simulink model "cessna_practicemodel"  (R2022a)
settings: Solver=VariableStepAuto  StartTime=0.0  StopTime=10  RelTol=1e-3
undefined symbols (not defined in the file or in its folder): Clat, Clong, DiscIntNeverNeededParam, Kr, Kr_lat, krlat, krlong, Kw, Kw_lat, Kx, Kx_lat, kxlat, kxlong
libraries: airlib x1
settings Model: Creator=steph  LastModifiedBy=steph

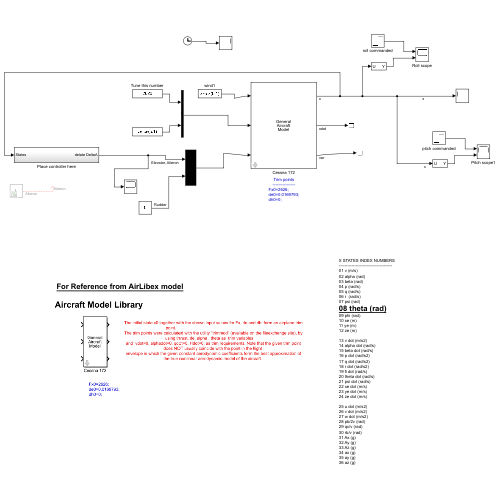
[thumbnail: Simulink's stored preview of the top-level diagram]
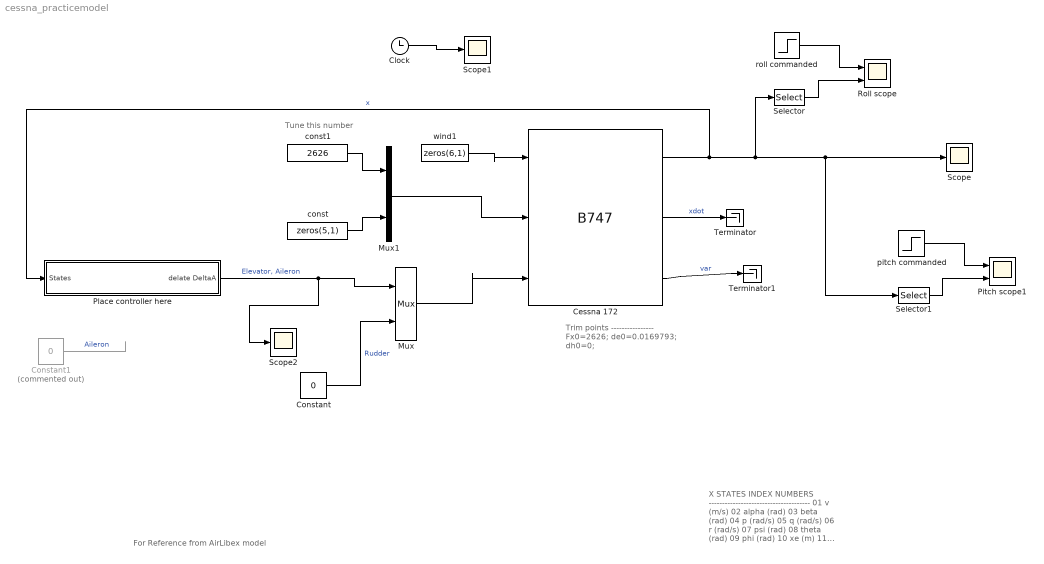
== system cessna_practicemodel ==
  note: For Reference from AirLibex model
  note: X STATES INDEX NUMBERS
      | --------------------------------------
      | 01 v (m/s)
      | 02 alpha (rad)
      | 03 beta (rad)
      | 04 p (rad/s)
      | 05 q (rad/s)
      | 06 r (rad/s)
      | 07 psi (rad)
      | 08 theta (rad)
      | 09 phi (rad)
      | 10 xe (m)
      | 11 ye (m)
      | 12 ze (m)
      |
      | 13 v dot (m/s2)
      | 14 alpha dot (rad/s)
      | 15 beta dot (rad/s)
      | 16 p dot (rad/s2)
      | 17 q dot (rad/s2)
      | 18 r dot (rad/s2)
      | 19 fi dot (rad/s)
      | 20 theta dot (rad/s)
      | 21 psi dot (rad/s)
      | 22 xe dot (m/s)
      | 23 ye dot (m/s)
      | 24 ze dot (m/s)
      |
      | 25 u dot (m/s2)
      | 26 v dot (m/s2)
      | 27 w dot (m/s2)
      | 28 pb/2v (rad)
      | 29 qc/v (rad)
      | 30 rb/v (rad)
      | 31 Ax (g)
      | 32 Ay (g)
      | 33 Az (g)
      | 34 ax (g)
      | 35 ay (g)
      | 36 az (g)
  note: Trim points
      | ----------------
      | Fx0=2626;
      | de0=0.0169793;
      | dh0=0;
  note: Tune this number
  " Cessna 172 " : airlib/B747  GM1="[1.4935  10.9118  16.1651  1285.3  1824.9  2666.9  0 0 0   1043.3]"  CD_wind="[0.031   0.13  0  0.06  0]"  CL_wind="[0.31   5.143    3.9   0.43   0]"  Cm_body="[-0.015  -0.89  -12.4   -1.28   0]"  CY_body="[0  -0.31 -0.037  0.21  0.0  0.187]"  Cl_body="[0    -0.089  -0.47  0.096  -0.178  0.0147]"  Cn_body="[0    0.065    -0.03  -0.099  -0.053  -0.0657]"  x0="[100  -0.0412737 0   0 0 0   0 -0.0412737 0   0 0 60]"
  Clock : Clock
  Constant : Constant  Value=0
  Constant1 : Constant  Commented=on  Value=0
  Mux : Mux  Inputs=2
  Mux1 : Mux  Inputs=[1 5]
  Pitch scope1 : Scope  NumInputPorts=2
  Place controller here : Subsystem
  Roll scope : Scope  NumInputPorts=2
  Scope : Scope
  Scope1 : Scope
  Scope2 : Scope
  Selector : Selector  InputPortWidth=12  IndexOptions=Index vector (dialog)  Indices=[9]  OutputSizes=1
  Selector1 : Selector  InputPortWidth=12  IndexOptions=Index vector (dialog)  Indices=[8]  OutputSizes=1
  Terminator : Terminator
  Terminator1 : Terminator
  const : Constant  Value=zeros(5,1)
  const1 : Constant  Value=2626
  pitch commanded : Step  Time=70  After=15*pi/180  SampleTime=0
  roll commanded : Step  Time=10  After=15*pi/180  SampleTime=0
  wind1 : Constant  Value=zeros(6,1)
  wires:
  " Cessna 172 "/2 -> Terminator/1  "xdot"
  " Cessna 172 "/3 -> Terminator1/1  "var"
  wind1/1 -> " Cessna 172 "/1
  Mux1/1 -> " Cessna 172 "/2
  Mux/1 -> " Cessna 172 "/3
  Place controller here/1(delate DeltaA) -> Scope2/1, Mux/1  "Elevator, Aileron"
  Constant/1 -> Mux/2  "Rudder"
  Constant1/1 -> ?  "Aileron"
  const/1 -> Mux1/2
  const1/1 -> Mux1/1
  Selector/1 -> Roll scope/2
  roll commanded/1 -> Roll scope/1
  " Cessna 172 "/1 -> Place controller here/1(States), Selector/1, Selector1/1, Scope/1  "x"
  Selector1/1 -> Pitch scope1/2
  pitch commanded/1 -> Pitch scope1/1
  Clock/1 -> Scope1/1

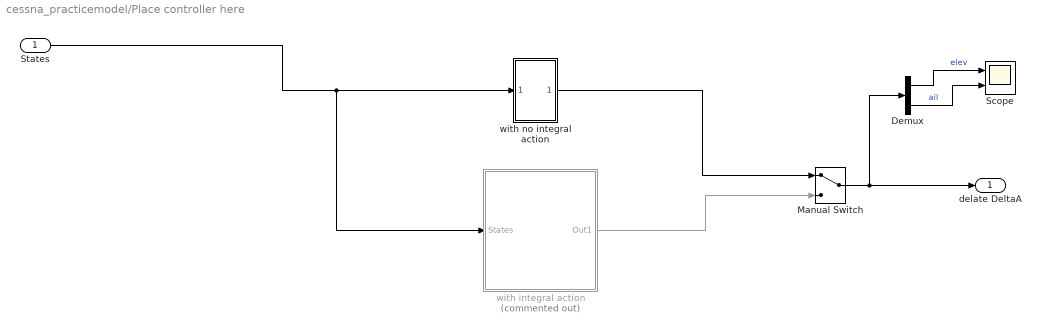
== system cessna_practicemodel/Place controller here ==
  States : Inport
  Demux : Demux  Outputs=2
  Manual Switch : ManualSwitch
  Scope : Scope  NumInputPorts=2
  with integral action : Subsystem  Commented=on
  with no integral action : Subsystem
  delate DeltaA : Outport
  wires:
  States/1 -> with integral action/1(States), with no integral action/1(In1)
  Manual Switch/1 -> Demux/1, delate DeltaA/1
  with no integral action/1(Out1) -> Manual Switch/1
  with integral action/1(Out1) -> Manual Switch/2
  Demux/1 -> Scope/1  "elev"
  Demux/2 -> Scope/2  "ail"

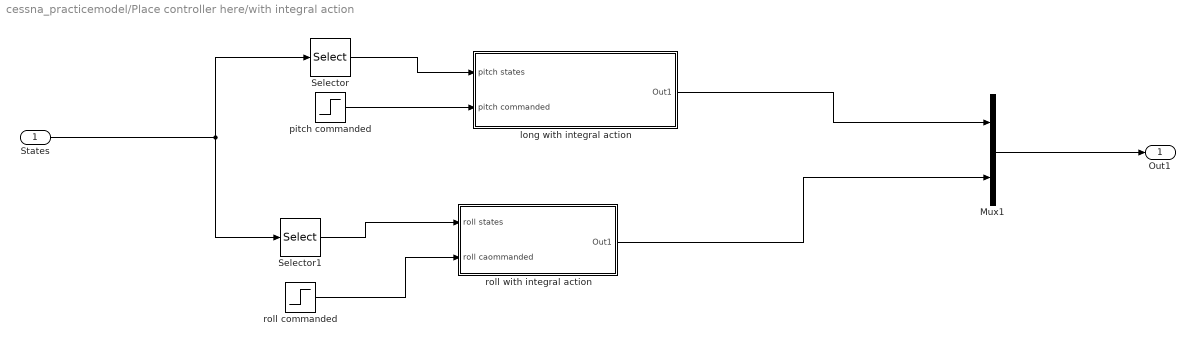
== system cessna_practicemodel/Place controller here/with integral action ==
  States : Inport
  Mux1 : Mux  Inputs=[1 2]
  Selector : Selector  InputPortWidth=12  IndexOptions=Index vector (dialog)  Indices=[1 2 5 8]  OutputSizes=1
  Selector1 : Selector  InputPortWidth=12  IndexOptions=Index vector (dialog)  Indices=[3 4 6 9]  OutputSizes=1
  long with integral action : Subsystem
  pitch commanded : Step  Time=70  After=15*pi/180  SampleTime=0
  roll commanded : Step  Time=10  After=15*pi/180  SampleTime=0
  roll with integral action : Subsystem
  Out1 : Outport
  wires:
  States/1 -> Selector1/1, Selector/1
  pitch commanded/1 -> long with integral action/2(pitch commanded)
  Selector/1 -> long with integral action/1(pitch states)
  roll commanded/1 -> roll with integral action/2(roll caommanded)
  Selector1/1 -> roll with integral action/1(roll states)
  Mux1/1 -> Out1/1
  roll with integral action/1(Out1) -> Mux1/2
  long with integral action/1(Out1) -> Mux1/1

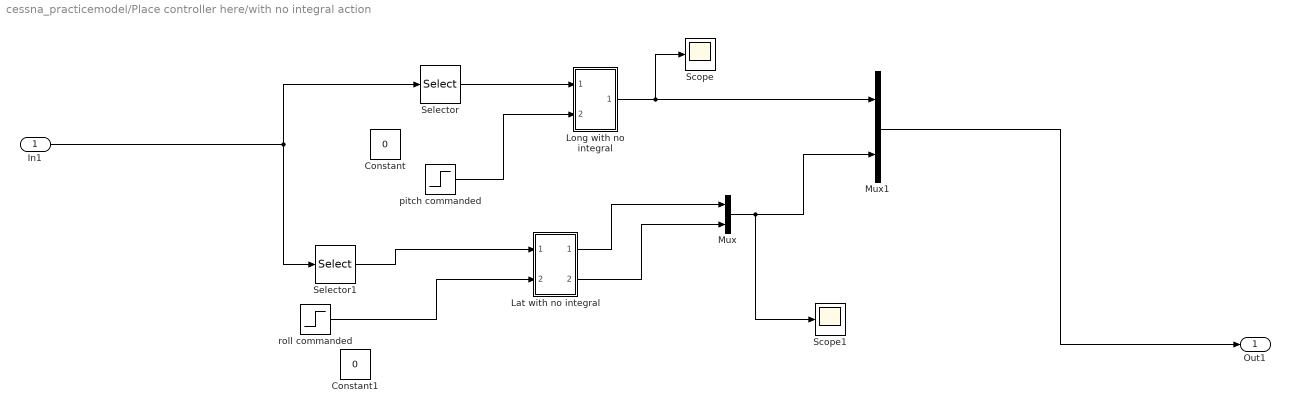
== system cessna_practicemodel/Place controller here/with no integral action ==
  In1 : Inport
  Constant : Constant  Value=0
  Constant1 : Constant  Value=0
  Lat with no integral : Subsystem
  Long with no integral : Subsystem
  Mux : Mux  Inputs=2
  Mux1 : Mux  Inputs=[1 2]
  Scope : Scope
  Scope1 : Scope
  Selector : Selector  InputPortWidth=12  IndexOptions=Index vector (dialog)  Indices=[1 2 5 8]  OutputSizes=1
  Selector1 : Selector  InputPortWidth=12  IndexOptions=Index vector (dialog)  Indices=[3 4 6 9]  OutputSizes=1
  pitch commanded : Step  Time=70  After=15*pi/180  SampleTime=0
  roll commanded : Step  Time=10  After=15*pi/180  SampleTime=0
  Out1 : Outport
  wires:
  Selector1/1 -> Lat with no integral/1(In1)
  Mux/1 -> Scope1/1, Mux1/2
  Selector/1 -> Long with no integral/1(In1)
  Lat with no integral/2(Out2) -> Mux/2
  Mux1/1 -> Out1/1
  Lat with no integral/1(Out1) -> Mux/1
  In1/1 -> Selector1/1, Selector/1
  pitch commanded/1 -> Long with no integral/2(In2)
  roll commanded/1 -> Lat with no integral/2(In2)
  Long with no integral/1(Out1) -> Mux1/1, Scope/1

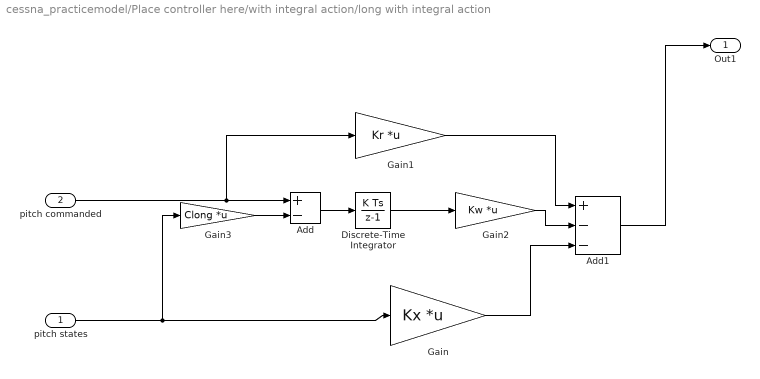
== system cessna_practicemodel/Place controller here/with integral action/long with integral action ==
  pitch states : Inport
  pitch commanded : Inport  Port=2
  Add : Sum  Inputs=+-
  Add1 : Sum  Inputs=+--
  Discrete-Time Integrator : DiscreteIntegrator  SampleTime=-1  ICPrevOutput=DiscIntNeverNeededParam  ICPrevScaledInput=DiscIntNeverNeededParam
  Gain : Gain  Gain=Kx  Multiplication=Matrix(K*u)
  Gain1 : Gain  Gain=Kr  Multiplication=Matrix(K*u)
  Gain2 : Gain  Gain=Kw  Multiplication=Matrix(K*u)
  Gain3 : Gain  Gain=Clong  Multiplication=Matrix(K*u)
  Out1 : Outport
  wires:
  pitch states/1 -> Gain3/1, Gain/1
  pitch commanded/1 -> Gain1/1, Add/1
  Add/1 -> Discrete-Time Integrator/1
  Discrete-Time Integrator/1 -> Gain2/1
  Gain1/1 -> Add1/1
  Gain2/1 -> Add1/2
  Gain/1 -> Add1/3
  Add1/1 -> Out1/1
  Gain3/1 -> Add/2

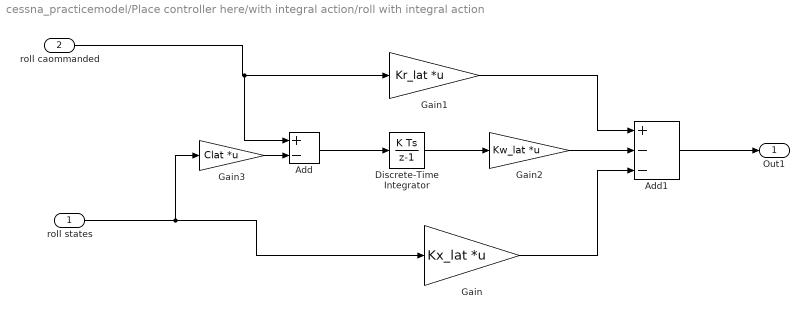
== system cessna_practicemodel/Place controller here/with integral action/roll with integral action ==
  roll states : Inport
  roll caommanded : Inport  Port=2
  Add : Sum  Inputs=+-
  Add1 : Sum  Inputs=+--
  Discrete-Time Integrator : DiscreteIntegrator  SampleTime=-1  ICPrevOutput=DiscIntNeverNeededParam  ICPrevScaledInput=DiscIntNeverNeededParam
  Gain : Gain  Gain=Kx_lat  Multiplication=Matrix(K*u)
  Gain1 : Gain  Gain=Kr_lat  Multiplication=Matrix(K*u)
  Gain2 : Gain  Gain=Kw_lat  Multiplication=Matrix(K*u)
  Gain3 : Gain  Gain=Clat  Multiplication=Matrix(K*u)
  Out1 : Outport
  wires:
  Gain/1 -> Add1/3
  Gain2/1 -> Add1/2
  Gain1/1 -> Add1/1
  roll states/1 -> Gain/1, Gain3/1
  Add1/1 -> Out1/1
  roll caommanded/1 -> Add/1, Gain1/1
  Add/1 -> Discrete-Time Integrator/1
  Discrete-Time Integrator/1 -> Gain2/1
  Gain3/1 -> Add/2

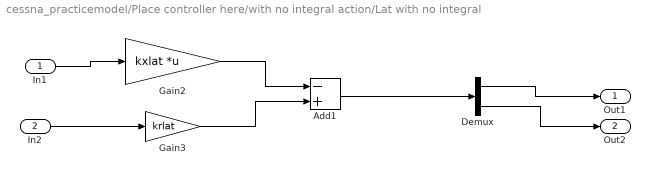
== system cessna_practicemodel/Place controller here/with no integral action/Lat with no integral ==
  In1 : Inport
  In2 : Inport  Port=2
  Add1 : Sum  Inputs=-+
  Demux : Demux  Outputs=2
  Gain2 : Gain  Gain=kxlat  Multiplication=Matrix(K*u)
  Gain3 : Gain  Gain=krlat
  Out1 : Outport
  Out2 : Outport  Port=2
  wires:
  Gain3/1 -> Add1/2
  Gain2/1 -> Add1/1
  In2/1 -> Gain3/1
  In1/1 -> Gain2/1
  Add1/1 -> Demux/1
  Demux/1 -> Out1/1
  Demux/2 -> Out2/1

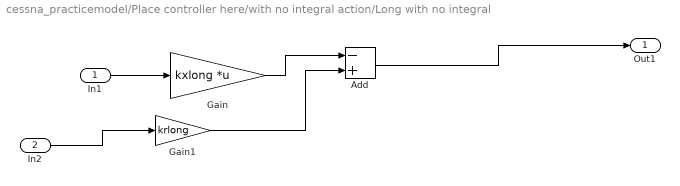
== system cessna_practicemodel/Place controller here/with no integral action/Long with no integral ==
  In1 : Inport
  In2 : Inport  Port=2
  Add : Sum  Inputs=-+
  Gain : Gain  Gain=kxlong  Multiplication=Matrix(K*u)
  Gain1 : Gain  Gain=krlong
  Out1 : Outport
  wires:
  Gain/1 -> Add/1
  Gain1/1 -> Add/2
  Add/1 -> Out1/1
  In1/1 -> Gain/1
  In2/1 -> Gain1/1
